simulink model "Bitchplzwork"  (Simulink 9.3)
settings: Solver=VariableStepAuto  StartTime=0.0  StopTime=1  FixedStep=0.1
values from neighbouring files (symbols this model uses):
  C = 13.5e-4    (= 0.00135)    [inverter.m]
  L = 27e-3    (= 0.027)    [inverter.m]
  R = 0.001    [inverter.m]
  Tss = 2.5e-6    (= 2.5e-06)    [inverter.m]
undefined symbols (not defined in the file or in its folder): Acid, Hydride, Lead, Metal, Nickel
libraries: powerlib x39, powerlib_extras x9, simulink x6, powerlib_meascontrol x4, electricdrivelib x2, re_lib x2, dsparch4 x1
(part 1 of 2)
settings Model: Creator=DELL  LastModifiedBy=DELL
settings Model: SuppressorTable=|
  | <?xml version="1.0" encoding="UTF-8" standalone="yes" ?>
  | <!DOCTYPE boost_serialization>
  | <boost_serialization signature="serialization::archive" version="15">
  | <DiagnosticSuppressor class_id="0" tracking_level="0" version="6">
  | 	<Table class_id="1" tracking_level="0" version="0">
  | 		<count>3</count>
  | 		<bucket_count>8</bucket_count>
  | 		<item_version>0</item_version>
  | 		<item class_id="2" tracking_level="0" version="0">
  | 			<first class_id="3" tracking_level="0" version="6">
  | 				<Source class_id="4" tracking_level="0" version="0">
  | 					<count>1</count>
  | 					<item_version>0</item_version>
  | 					<item>Bitchplzwork/PV array 1/irradiation /LimitedCounter</item>
  | 				</Source>
  | 			</first>
  | 			<second class_id="5" tracking_level="0" version="6">
  | 				<SuppressedData class_id="6" tracking_level="0" version="0">
  | 					<count>2</count>
  | 					<bucket_count>8</bucket_count>
  | 					<item_version>0</item_version>
  | 					<item class_id="7" tracking_level="0" version="0">
  | 						<first class_id="8" tracking_level="0" version="6">
  | 							<ID>Simulink:DataType:WarningOverFlowDetected</ID>
  | 							<Cause>
  | 								<Source>
  | 									<count>0</count>
  | 									<item_version>0</item_version>
  | 								</Source>
  | 							</Cause>
  | 						</first>
  | 						<second class_id="9" tracking_level="0" version="6">
  | 							<Comment></Comment>
  | 							<User></User>
  | 							<LastModified class_id="10" tracking_level="0" version="0">
  | 								<ptime_date class_id="11" tracking_level="0" version="0">
  | 									<date>20160608</date>
  | 								</ptime_date>
  | 								<ptime_time_duration class_id="12" tracking_level="0" version="0">
  | 									<is_special>0</is_special>
  | 									<time_duration_hours>15</time_duration_hours>
  | 									<time_duration_minutes>23</time_duration_minutes>
  | 									<time_duration_seconds>17</time_duration_seconds>
  | 									<time_duration_fractional_seconds>0</time_duration_fractional_seconds>
  | 								</ptime_time_duration>
  | 							</LastModified>
  | 							<SuppressionType>1</SuppressionType>
  | 						</second>
  | 					</item>
  | 					<item>
  | 						<first>
  | 							<ID>SimulinkFixedPoint:util:Overflowoccurred</ID>
  | 							<Cause>
  | 								<Source>
  | 									<count>0</count>
  | 									<item_version>0</item_version>
  | 								</Source>
  | 							</Cause>
  | 						</first>
  | 						<second>
  | 							<Comment></Comment>
  | 							<User></User>
  | 							<LastModified>
  | 								<ptime_date>
  | 									<date>20160608</date>
  | 								</ptime_date>
  | 								<ptime_time_duration>
  | 									<is_special>0</is_special>
  | 									<time_duration_hours>15</time_duration_hours>
  | 									<time_duration_minutes>23</time_duration_minutes>
  | 									<time_duration_seconds>17</time_duration_seconds>
  | 									<time_duration_fractional_seconds>0</time_duration_fractional_seconds>
  | 								</ptime_time_duration>
  | 							</LastModified>
  | 							<SuppressionType>1</SuppressionType>
  | 						</second>
  | 					</item>
  | 				</SuppressedData>
  | 			</second>
  | 		</item>
  | 		<item>
  | 			<first>
  | 				<Source>
  | 					<count>1</count>
  | 					<item_version>0</item_version>
  | 					<item>Bitchplzwork/PV array 1/Temperature/LimitedCounter</item>
  | 				</Source>
  | 			</first>
  | 			<second>
  | 				<SuppressedData>
  | 					<count>2</count>
  | 					<bucket_count>8</bucket_count>
  | 					<item_version>0</item_version>
  | 					<item>
  | 						<first>
  | 							<ID>Simulink:DataType:WarningOverFlowDetected</ID>
  | 							<Cause>
  | 								<Source>
  | 									<count>0</count>
  | 									<item_version>0</item_version>
  | 								</Source>
  | 							</Cause>
  | 						</first>
  | 						<second>
  | 							<Comment></Comment>
  | 							<User></User>
  | 							<LastModified>
  | 								<ptime_date>
  | 									<date>20160608</date>
  | 								</ptime_date>
  | 								<ptime_time_duration>
  | 									<is_special>0</is_special>
  | 									<time_duration_hours>15</time_duration_hours>
  | 									<time_duration_minutes>23</time_duration_minutes>
  | 									<time_duration_seconds>17</time_duration_seconds>
  | 									<time_duration_fractional_seconds>0</time_duration_fractional_seconds>
  | 								</ptime_time_duration>
  | 							</LastModified>
  | 							<SuppressionType>1</SuppressionType>
  | 						</second>
  | 					</item>
  | 					<item>
  | 						<first>
  | 							<ID>SimulinkFixedPoint:util:Overflowoccurred</ID>
  | 							<Cause>
  | 								<Source>
  | 									<count>0</count>
  | 									<item_version>0</item_version>
  | 								</Source>
  | 							</Cause>
  | 						</first>
  | 						<second>
  | 							<Comment></Comment>
  | 							<User></User>
  | 							<LastModified>
  | 								<ptime_date>
  | 									<date>20160608</date>
  | 								</ptime_date>
  | 								<ptime_time_duration>
  | 									<is_special>0</is_special>
  | 									<time_duration_hours>15</time_duration_hours>
  | 									<time_duration_minutes>23</time_duration_minutes>
  | 									<time_duration_seconds>17</time_duration_seconds>
  | 									<time_duration_fractional_seconds>0</time_duration_fractional_seconds>
  | 								</ptime_time_duration>
  | 							</LastModified>
  | 							<SuppressionType>1</SuppressionType>
  | 						</second>
  | 					</item>
  | 				</SuppressedData>
  | 			</second>
  | 		</item>
  | 		<item>
  | 			<first>
  | 				<Source>
  | 					<count>1</count>
  | 					<item_version>0</item_version>
  | 					<item>Bitchplzwork/Wind 3 KW, 50HZ, 440V1/Wind Speed/LimitedCounter</item>
  | 				</Source>
  | 			</first>
  | 			<second>
  | 				<SuppressedData>
  | 					<count>2</count>
  | 					<bucket_count>8</bucket_count>
  | 					<item_version>0</item_version>
  | 					<item>
  | 						<first>
  | 							<ID>Simulink:DataType:WarningOverFlowDetected</ID>
  | 							<Cause>
  | 								<Source>
  | 									<count>0</count>
  | 									<item_version>0</item_version>
  | 								</Source>
  | 							</Cause>
  | 						</first>
  | 						<second>
  | 							<Comment></Comment>
  | 							<User></User>
  | 							<LastModified>
  | 								<ptime_date>
  | 									<date>20160608</date>
  | 								</ptime_date>
  | 								<ptime_time_duration>
  | 									<is_special>0</is_special>
  | 									<time_duration_hours>15</time_duration_hours>
  | 									<time_duration_minutes>23</time_duration_minutes>
  | 									<time_duration_seconds>17</time_duration_seconds>
  | 									<time_duration_fractional_seconds>0</time_duration_fractional_seconds>
  | 								</ptime_time_duration>
  | 							</LastModified>
  | 							<SuppressionType>1</SuppressionType>
  | 						</second>
  | 					</item>
  | 					<item>
  | 						<first>
  | 							<ID>SimulinkFixedPoint:util:Overflowoccurred</ID>
  | 							<Cause>
  | 								<Source>
  | 									<count>0</count>
  | 									<item_version>0</item_version>
  | 								</Source>
  | 							</Cause>
  | 						</first>
  | 						<second>
  | 							<Comment></Comment>
  | 							<User></User>
  | 							<LastModified>
  | 								<ptime_date>
  | 									<date>20160608</date>
  | 								</ptime_date>
  | 								<ptime_time_duration>
  | 									<is_special>0</is_special>
  | 									<time_duration_hours>15</time_duration_hours>
  | 									<time_duration_minutes>23</time_duration_minutes>
  | 									<time_duration_seconds>17</time_duration_seconds>
  | 									<time_duration_fractional_seconds>0</time_duration_fractional_seconds>
  | 								</ptime_time_duration>
  | 							</LastModified>
  | 							<SuppressionType>1</SuppressionType>
  | 						</second>
  | 					</item>
  | 				</SuppressedData>
  | 			</second>
  | 		</item>
  | 	</Table>
  | </DiagnosticSuppressor>
  | </boost_serialization>
settings DataIOCC: SaveFormat=Dataset  SignalLoggingSaveFormat=Dataset  ReturnWorkspaceOutputs=on
settings OptimizationCC: LifeSpan=auto
settings DebuggingCC: UnderspecifiedInitializationDetection=Simplified  MergeDetectMultiDrivingBlocksExec=error  FcnCallInpInsideContextMsg=error  SFUnexpectedBacktrackingDiag=error  SFNoUnconditionalDefaultTransitionDiag=error  SFExecutionAtInitializationDiag=warning  ArithmeticOperatorsInVariantConditions=error
settings HardwareCC: ProdBitPerPointer=64  ProdBitPerSizeT=64  ProdBitPerPtrDiffT=64  ProdLargestAtomicFloat=Float  ProdIntDivRoundTo=Zero  ProdEndianess=LittleEndian  ProdWordSize=64  ProdHWDeviceType=Intel->x86-64 (Windows64)
settings ModelReferenceCC: PropagateSignalLabelsOutOfModel=on
settings SFSimCC: SimUseLocalCustomCode=on
settings RTWCC: RTWUseLocalCustomCode=on
settings CodeAppCC: StateflowObjectComments=off
settings GRTTargetCC: TargetLangStandard=C99 (ISO)  CombineOutputUpdateFcns=on  GRTInterface=off
settings ConfigComp: CovMetricSettings=dwe  CovHtmlReporting=off  CovSaveCumulativeToWorkspaceVar=off  CovSaveSingleToWorkspaceVar=off  CovExternalEMLEnable=on

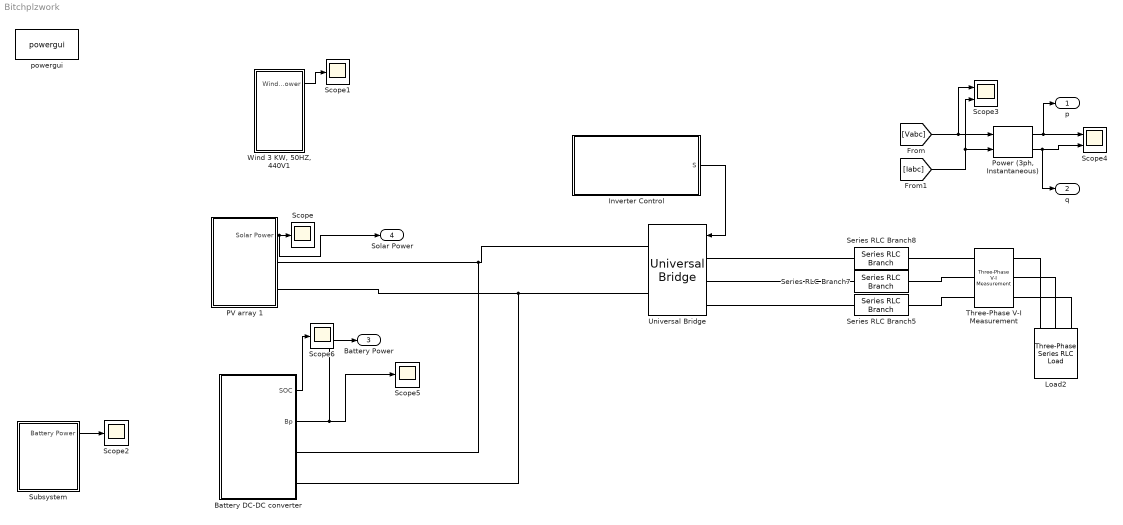
== system Bitchplzwork ==
  "Battery DC-DC converter " : Subsystem
  Inverter Control : Subsystem
  Load2 : powerlib/Elements/Three-Phase Series RLC Load  LConnTagsString=A|B|C  Configuration=Y (grounded)  NominalVoltage=400  Vabc=[1e3 1e3 1e3]  Vabcp=[1e3 1e3 1e3]  NominalFrequency=50  UnbalancedPower=off  ActivePower=400e3  InductivePower=0  CapacitivePower=0  Pabc=[10e3 9e3 11e3]  QLabc=[100 90 110]  QCabc=[100 90 110]  Pabcp=[10e3 9e3 11e3]  QLabcp=[100 90 110]  QCabcp=[100 90 110]  Measurements=None  LoadType=constant Z
      settings: SourceProductName=Simscape Electrical
  PV array 1 : Subsystem
  "Power (3ph, Instantaneous)" : powerlib_meascontrol/Measurements/Power (3ph, Instantaneous)
      settings: SourceProductName=Simscape Electrical
  Scope{,1..2,5..6} (5 alike) : Scope
  Scope3 : Scope  NumInputPorts=2
  Scope4 : Scope  NumInputPorts=2
  Series RLC Branch5 : powerlib/Elements/Series RLC Branch  LConnTagsString=__new0  RConnTagsString=__new0  BranchType=LC  Resistance=R  Inductance=L  SetiL0=off  InitialCurrent=0  Capacitance=C  Setx0=off  InitialVoltage=0  Measurements=Branch voltage
      settings: SourceProductName=Simscape Electrical
  Series RLC Branch7 : powerlib/Elements/Series RLC Branch  LConnTagsString=__new0  RConnTagsString=__new0  BranchType=LC  Resistance=R  Inductance=L  SetiL0=off  InitialCurrent=0  Capacitance=C  Setx0=off  InitialVoltage=0  Measurements=Branch voltage
      settings: SourceProductName=Simscape Electrical
  Series RLC Branch8 : powerlib/Elements/Series RLC Branch  LConnTagsString=__new0  RConnTagsString=__new0  BranchType=LC  Resistance=R  Inductance=L  SetiL0=off  InitialCurrent=0  Capacitance=C  Setx0=off  InitialVoltage=0  Measurements=Branch voltage
      settings: SourceProductName=Simscape Electrical
  Subsystem : Subsystem
  Three-Phase V-I Measurement : powerlib/Measurements/Three-Phase V-I Measurement  VoltageMeasurement=phase-to-ground  SetLabelV=on  LabelV=Vabc  Vpu=off  VpuLL=off  CurrentMeasurement=yes  SetLabelI=on  LabelI=Iabc  Ipu=off  Pbase=100e6  Vbase=500e3  OutputType=Complex  PhasorSimulation=off  PSBequivalent=0
      settings: SourceProductName=Simscape Electrical
  Universal Bridge : powerlib/Power Electronics/Universal Bridge  Arms=3  SnubberResistance=1e5  SnubberCapacitance=inf  Device=IGBT / Diodes  Ron=1e-3  Lon=0  ForwardVoltages="[  0  0  ]"  ForwardVoltage=0  GTOparameters=[ 10e-6 , 20e-6 ]  IGBTparameters=[ 1e-6 , 2e-6 ]  Measurements=None  Measurements_2=None  converterType=Rectifier
      settings: SourceProductName=Simscape Electrical
  "Wind 3 KW, 50HZ, 440V1" : Subsystem
  powergui : powerlib/powergui  Priority=1  SimulationMode=Continuous  SampleTime=Tss  frequency=60  Iterations=50  frequencyindice=0  Pbase=100e6  ErrMax=1e-4  UnitsV=kV  UnitsW=MW  buscounter=0  FunctionMessages=off  echomessages=off  EnableUseOfTLC=off  CurrentSourceSwitches=off  DisableSnubberDevices=off  DisableRonSwitches=off  DisableVfSwitches=off  DisplayEquations=off  AutomaticDiscreteSolvers=off  SolverType=Tustin/Backward Euler (TBE)  Interpol=off  ExternalGateDelay=off  methode=off  Ts=100  x0status=blocks  SPID=on  SwTol=0  HookPort=off  NonlinearTolerance=0  nMaxIteration=15  ContinueOnMaxIteration=off  RestoreLinks=warning  ResistiveCurrentMeasurement=off  Frange=[0:2:500]  Ylog=off  Xlog=on  ShowGrid=off  save=off  variable=ZData  structure=0  ZoomFFT=off  StartTime=0.0  cycles=1  DisplayStyle=1  fundamental=60  FreqAxis=off  MaxFrequency=1000  frequencyindicesteady=1  RmsSteady=1  display=off
      settings: SourceProductName=Simscape Electrical
  p : Outport
  q : Outport  Port=2
  Battery Power : Outport  Port=3
  Solar Power : Outport  Port=4
  wires:
  PV array 1/1(Solar Power) -> Solar Power/1, Scope/1
  "Wind 3 KW, 50HZ, 440V1"/1(Wind Power) -> Scope1/1
  Subsystem/1("Battery Power ") -> Scope2/1
  "Power (3ph, Instantaneous)"/2 -> q/1, Scope4/2
  "Power (3ph, Instantaneous)"/1 -> Scope4/1, p/1
  [Vabc] -> Scope3/1, "Power (3ph, Instantaneous)"/1
  [Iabc] -> Scope3/2, "Power (3ph, Instantaneous)"/2
  Inverter Control/1(S) -> Universal Bridge/1
  "Battery DC-DC converter "/2(Bp) -> Battery Power/1, Scope5/1
  "Battery DC-DC converter "/1(SOC) -> Scope6/1
  connections:
  PV array 1/RConn1 -- "Battery DC-DC converter "/RConn1 -- Universal Bridge/RConn1
  PV array 1/RConn2 -- "Battery DC-DC converter "/RConn2 -- Universal Bridge/RConn2
  Three-Phase V-I Measurement/LConn1 -- Series RLC Branch8/RConn1
  Series RLC Branch7/RConn1 -- Three-Phase V-I Measurement/LConn2
  Series RLC Branch5/RConn1 -- Three-Phase V-I Measurement/LConn3
  Three-Phase V-I Measurement/RConn1 -- Load2/LConn1
  Three-Phase V-I Measurement/RConn2 -- Load2/LConn2
  Three-Phase V-I Measurement/RConn3 -- Load2/LConn3
  Universal Bridge/LConn1 -- Series RLC Branch8/LConn1
  Universal Bridge/LConn2 -- Series RLC Branch7/LConn1
  Universal Bridge/LConn3 -- Series RLC Branch5/LConn1

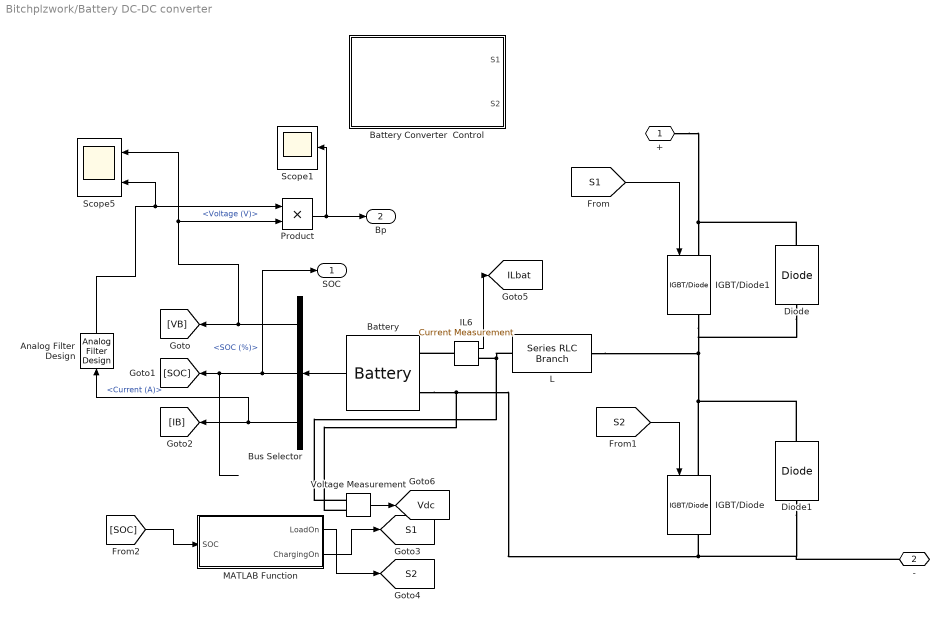
== system Bitchplzwork/Battery DC-DC converter  ==
  Analog Filter Design : dsparch4/Analog Filter Design  method=Butterworth  filttype=Lowpass  N=8  Wlo=30  Whi=80  Rp=2  Rs=40
  Battery : electricdrivelib/Extra Sources/Battery  BatType=Lead-Acid  ShowTempParam=off  ThermalPreset=no  ShowAgeParam=off  NomV=250  NomQ=500  SOC=80  Batt_Tr=30  PresetModel=on  MaxQ=520.8333  MinV=187.5  FullV=272.2039  Dis_rate=100  R=0.005  Normal_OP=155.1389  expZone="[254.523      1.666667]"  current=[6.5 13 32.5]  Units=Time  Tci=20  NomT=20  T2=-30  MaxQ2=4.8  FullV2=7.1  Normal_OP2=5.655  expZone2="[6.58           1]"  Rca=0.6  ti=2000  Dp=0  Neq0=0  Tsim=1e6  Ta1=25  Qeol=5.4*0.9  Reol=0.013333*1.2  Char_age=[2.3478, 3]  Dis_age=[2.3478, 10]  N1=1500  N2=10500  N3=1000  N4=1400  Ta2=45  N5=950
      settings: SourceProductName=Simscape Electrical
  Battery Converter  Control : Subsystem
  Bus Selector : BusSelector  OutputSignals=Voltage (V),SOC (%),Current (A)
  Diode : powerlib/Power Electronics/Diode  Ron=0.001  Lon=0  Vf=0.8  IC=0  UseSnubber=0  Rs=500  Cs=250e-9  Measurements=off
      settings: SourceProductName=Simscape Electrical
  Diode1 : powerlib/Power Electronics/Diode  Ron=0.001  Lon=0  Vf=0.8  IC=0  UseSnubber=0  Rs=500  Cs=250e-9  Measurements=off
      settings: SourceProductName=Simscape Electrical
  IGBT/Diode : powerlib/Power Electronics/IGBT//Diode  Ron=1e-3  Rs=1e5  Cs=inf  Measurements=on
      settings: SourceProductName=Simscape Electrical
  IGBT/Diode1 : powerlib/Power Electronics/IGBT//Diode  Ron=1e-3  Rs=1e5  Cs=inf  Measurements=on
      settings: SourceProductName=Simscape Electrical
  IL6 : powerlib/Measurements/Current Measurement  PhasorSimulation=off  OutputType=Complex  PSBequivalent=0
      settings: SourceProductName=Simscape Electrical
  L : powerlib/Elements/Series RLC Branch  LConnTagsString=__new0  RConnTagsString=__new0  BranchType=L  Resistance=0.1  Inductance=1e-3  SetiL0=off  InitialCurrent=0  Capacitance=1e-6  Setx0=off  InitialVoltage=0  Measurements=None
      settings: SourceProductName=Simscape Electrical
  MATLAB Function : MATLAB Function  TreatAsAtomicUnit=on
  Product : Product
  Scope1 : Scope
  Scope5 : Scope  NumInputPorts=2
  Voltage Measurement : powerlib/Measurements/Voltage Measurement  PhasorSimulation=off  OutputType=Complex  PSBequivalent=0
      settings: SourceProductName=Simscape Electrical
  + : PMIOPort  Side=Right
  - : PMIOPort  Port=2  Side=Right
  SOC : Outport
  Bp : Outport  Port=2
  tag scope: ILbat=global, S1=global, S2=global, Vdc=global
  wires:
  Bus Selector/1 -> [VB], Product/2, Scope5/1  "<Voltage (V)>"
  Product/1 -> Bp/1, Scope1/1
  Bus Selector/2 -> [SOC], SOC/1  "<SOC (%)>"
  Analog Filter Design/1 -> Scope5/2, Product/1
  Battery/1 -> Bus Selector/1
  Bus Selector/3 -> Analog Filter Design/1, [IB]  "<Current (A)>"
  [S2] -> IGBT/Diode/1
  [S1] -> IGBT/Diode1/1
  IL6/1 -> [ILbat]
  Voltage Measurement/1 -> [Vdc]
  [SOC] -> MATLAB Function/1(SOC)
  MATLAB Function/2(ChargingOn) -> [S1]
  MATLAB Function/1(LoadOn) -> [S2]
  connections:
  IL6/LConn1 -- Battery/LConn1
  Battery/LConn2 -- Voltage Measurement/LConn2 -- -/RConn1 -- Diode1/LConn1 -- IGBT/Diode/RConn1
  Diode/RConn1 -- +/RConn1 -- IGBT/Diode1/LConn1
  L/LConn1 -- Diode/LConn1 -- IGBT/Diode1/RConn1 -- Diode1/RConn1 -- IGBT/Diode/LConn1
  L/RConn1 -- Voltage Measurement/LConn1 -- IL6/RConn1

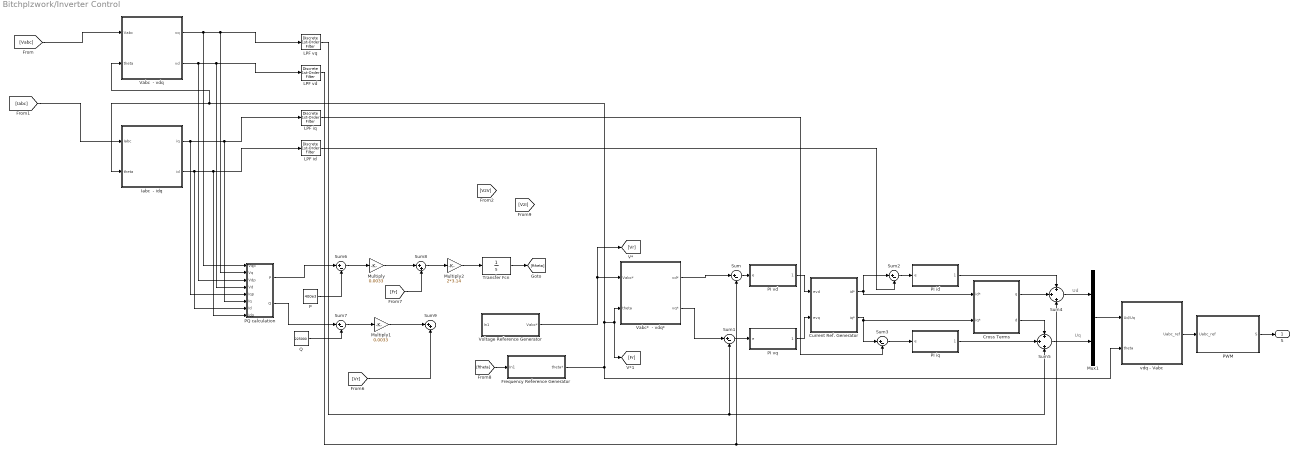
== system Bitchplzwork/Inverter Control ==
  note: Ud
  note: Uq
  " Voltage Reference Generator" : Subsystem
  Cross Terms : Subsystem
  Current Ref. Generator : Subsystem
  Frequency Reference Generator : Subsystem
  Iabc  - idq : Subsystem
  LPF id : powerlib_extras/Discrete  Control Blocks/Discrete 1st-Order Filter  FilterType=Lowpass  Tc=1e-3  Ts=5e-6  Initialize=off  Vac_Init=[0.8 -25 60]  Vdc_Init=0  PlotResponse=off  param1=[1 100 0.1]
      settings: SourceProductName=Simscape Electrical  SourceProductBaseCode=PS
  LPF iq : powerlib_extras/Discrete  Control Blocks/Discrete 1st-Order Filter  FilterType=Lowpass  Tc=1e-3  Ts=5e-6  Initialize=off  Vac_Init=[0.8 -25 60]  Vdc_Init=0  PlotResponse=off  param1=[1 100 0.1]
      settings: SourceProductName=Simscape Electrical  SourceProductBaseCode=PS
  LPF vd : powerlib_extras/Discrete  Control Blocks/Discrete 1st-Order Filter  FilterType=Lowpass  Tc=10e-3  Ts=5e-6  Initialize=off  Vac_Init=[0.8 -25 60]  Vdc_Init=-0.4  PlotResponse=off  param1=[1 100 0.1]
      settings: SourceProductName=Simscape Electrical  SourceProductBaseCode=PS
  LPF vq : powerlib_extras/Discrete  Control Blocks/Discrete 1st-Order Filter  FilterType=Lowpass  Tc=10e-3  Ts=5e-6  Initialize=off  Vac_Init=[0.8 -25 60]  Vdc_Init=0  PlotResponse=off  param1=[1 100 0.1]
      settings: SourceProductName=Simscape Electrical  SourceProductBaseCode=PS
  Multiply : Gain  Gain=0.0033
  Multiply1 : Gain  Gain=0.0033
  Multiply2 : Gain  Gain=2*3.14
  Mux1 : Mux  Inputs=2
  P : Constant  Value=400e3
  PI id : Subsystem
  PI iq : Subsystem
  PI vd : Subsystem
  PI vq : Subsystem
  PQ calculation : Subsystem
  PWM : Subsystem
  Q : Constant  Value=225000
  Sum{,1..3,6..7} (6 alike) : Sum  Inputs=|+-
  Sum4 : Sum  Inputs=+|+|+
  Sum5 : Sum  Inputs=+|+|+
  Sum8 : Sum  Inputs=|++
  Sum9 : Sum  Inputs=|++
  Transfer Fcn : TransferFcn  Denominator=[0 1 0]
  Vabc  - vdq : Subsystem
  Vabc*  - vdq* : Subsystem
  vdq - Vabc : Subsystem
  S : Outport
  wires:
  [Vabc] -> Vabc  - vdq/1(Vabc)
  [Iabc] -> Iabc  - idq/1(Iabc)
  Sum2/1 -> PI id/1(e)
  Sum3/1 -> PI iq/1(e)
  Mux1/1 -> vdq - Vabc/1(Ud/Uq)
  vdq - Vabc/1(Uabc_ref) -> PWM/1(Uabc_ref)
  PWM/1(S) -> S/1
  Vabc  - vdq/2(vd) -> PQ calculation/3(Vdp), PQ calculation/4(Vd), LPF vd/1
  Iabc  - idq/1(iq) -> PQ calculation/5(Iqp), PQ calculation/6(Iq), LPF iq/1
  Iabc  - idq/2(id) -> PQ calculation/7(Id), PQ calculation/8(Idq), LPF id/1
  LPF vd/1 -> Sum/2, Sum4/3
  LPF vq/1 -> Sum1/2, Sum5/3
  LPF iq/1 -> Sum3/2
  LPF id/1 -> Sum2/2
  Sum/1 -> PI vd/1(e)
  Sum1/1 -> PI vq/1(e)
  Vabc*  - vdq*/1(vd*) -> Sum/1
  Vabc*  - vdq*/2(vq*) -> Sum1/1
  Frequency Reference Generator/1(theta*) -> Vabc  - vdq/2(theta), Iabc  - idq/2(theta), [Fr], Vabc*  - vdq*/2(theta), vdq - Vabc/2(theta)
  PI vd/1(" ") -> Current Ref. Generator/1(evd)
  PI vq/1(" ") -> Current Ref. Generator/2(evq)
  Current Ref. Generator/2(iq*) -> Sum3/1, Cross Terms/2(iq*)
  Current Ref. Generator/1(id*) -> Cross Terms/1(id*), Sum2/1
  PI iq/1(" ") -> Sum5/2
  PI id/1(" ") -> Sum4/1
  Cross Terms/1(" q") -> Sum4/2
  Cross Terms/2(" d") -> Sum5/1
  Sum5/1 -> Mux1/2
  Sum4/1 -> Mux1/1
  Vabc  - vdq/1(vq) -> PQ calculation/1(Vqp), PQ calculation/2(Vq), LPF vq/1
  PQ calculation/1(P) -> Sum6/1
  P/1 -> Sum6/2
  Sum6/1 -> Multiply/1
  Q/1 -> Sum7/2
  PQ calculation/2(Q) -> Sum7/1
  Sum7/1 -> Multiply1/1
  Multiply/1 -> Sum8/1
  [Fr] -> Sum8/2
  Multiply1/1 -> Sum9/1
  [Vr] -> Sum9/2
  Sum8/1 -> Multiply2/1
  Multiply2/1 -> Transfer Fcn/1
  Transfer Fcn/1 -> [ftheta]
  [ftheta] -> Frequency Reference Generator/1(In1)
  " Voltage Reference Generator"/1(Vabc*) -> [Vr], Vabc*  - vdq*/1(Vabc*)

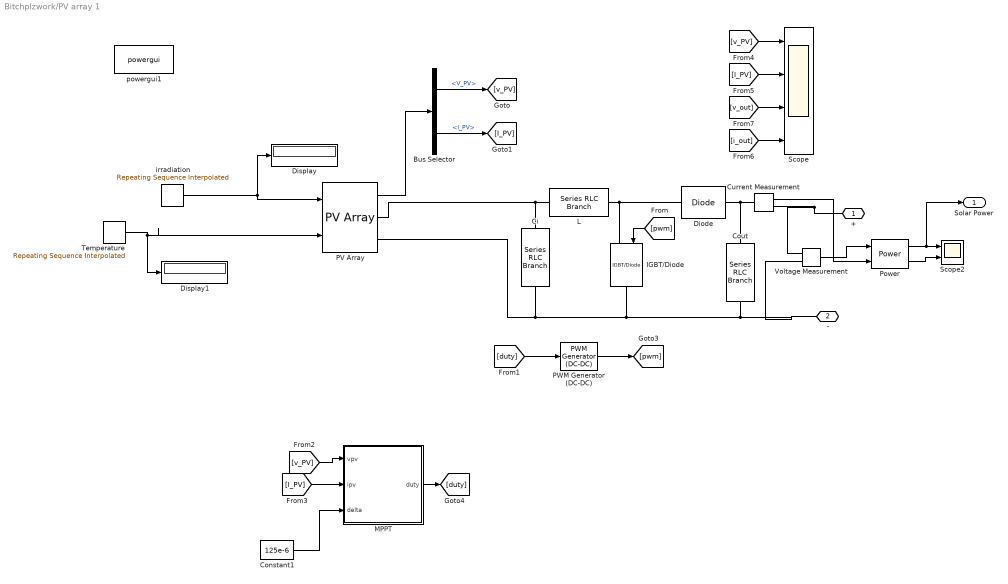
== system Bitchplzwork/PV array 1 ==
  Bus Selector : BusSelector  OutputSignals=V_PV,I_PV
  Ci : powerlib/Elements/Series RLC Branch  LConnTagsString=__new0  RConnTagsString=__new0  BranchType=RC  Resistance=1E-4  Inductance=1e-3  SetiL0=off  InitialCurrent=0  Capacitance=100E-6  Setx0=off  InitialVoltage=0  Measurements=None
      settings: SourceProductName=Simscape Electrical
  Constant1 : Constant  Value=125e-6
  Cout : powerlib/Elements/Series RLC Branch  LConnTagsString=__new0  RConnTagsString=__new0  BranchType=RC  Resistance=1E-4  Inductance=1e-3  SetiL0=off  InitialCurrent=0  Capacitance=100E-6  Setx0=off  InitialVoltage=0  Measurements=None
      settings: SourceProductName=Simscape Electrical
  Current Measurement : powerlib/Measurements/Current Measurement  PhasorSimulation=off  OutputType=Complex  PSBequivalent=0
      settings: SourceProductName=Simscape Electrical
  Diode : powerlib/Power Electronics/Diode  Ron=0.001  Lon=0  Vf=0.8  IC=0  UseSnubber=0  Rs=500  Cs=250e-9  Measurements=off
      settings: SourceProductName=Simscape Electrical
  Display : Display
  Display1 : Display
  IGBT/Diode : powerlib/Power Electronics/IGBT//Diode  Ron=1e-3  Rs=1e5  Cs=inf  Measurements=off
      settings: SourceProductName=Simscape Electrical
  L : powerlib/Elements/Series RLC Branch  LConnTagsString=__new0  RConnTagsString=__new0  BranchType=RL  Resistance=0.1  Inductance=2E-3  SetiL0=off  InitialCurrent=0  Capacitance=100E-6  Setx0=off  InitialVoltage=0  Measurements=None
      settings: SourceProductName=Simscape Electrical
  MPPT : MATLAB Function  TreatAsAtomicUnit=on
  PV Array : re_lib/Solar/PV Array  Npar=150  Nser=10  PlotType=array @ 1000 W/m2 & specified temperatures  S_vec="[ 1000  500  100 ]"  Temp_C_vec="[ 45 25  ]"  ModuleName=Shanghai JA Solar Technology JAP6-72-315-3BB  PlotWhenSelected=off  Pm=315.016  Ncell=72  Voc=46.42  Isc=8.74  Vm=37.28  Im=8.45  beta_Voc_pc=-0.3  alpha_Isc_pc=0.04  beta_Voc=-0.13926  alpha_Isc=0.003496  IL=8.9123  I0=3e-11  nI=0.95004  Rsh=1485.5559  Rs=0.45827  BAL=off  Tc=1e-6  Tfilter=5e-5
      settings: SourceProductName=Simscape Electrical
  PWM Generator (DC-DC) : powerlib_meascontrol/Pulse & Signal Generators/PWM Generator (DC-DC)  Fsw=5000  Ts=5e-6
      settings: SourceProductName=Simscape Electrical
  Power : powerlib_meascontrol/Measurements/Power  Freq=60  Vinit=[1, 0]  Iinit=[1, 0]  Ts=0
      settings: SourceProductName=Simscape Electrical
  Scope : Scope  NumInputPorts=4
  Scope2 : Scope  NumInputPorts=2
  Temperature : simulink/Sources/Repeating Sequence Interpolated  OutValues=temp  TimeValues=timeStamp  LookUpMeth=Interpolation-Use End Values  tsamp=0.1  OutMin=[]  OutMax=[]  OutDataTypeStr=double  OutputDataTypeScalingMode=double  OutDataType=fixdt(0,8)  OutScaling=2^-10
  Voltage Measurement : powerlib/Measurements/Voltage Measurement  PhasorSimulation=off  OutputType=Complex  PSBequivalent=0
      settings: SourceProductName=Simscape Electrical
  "irradiation " : simulink/Sources/Repeating Sequence Interpolated  OutValues=irrad  TimeValues=timeStamp  LookUpMeth=Interpolation-Use End Values  tsamp=0.1  OutMin=[]  OutMax=[]  OutDataTypeStr=double  OutputDataTypeScalingMode=double  OutDataType=fixdt(0,8)  OutScaling=2^-10
  powergui1 : powerlib/powergui  Priority=1  SimulationMode=Discrete  SampleTime=Tss  frequency=60  Iterations=50  frequencyindice=0  Pbase=100e6  ErrMax=1e-4  UnitsV=kV  UnitsW=MW  buscounter=0  FunctionMessages=off  echomessages=off  EnableUseOfTLC=off  CurrentSourceSwitches=off  DisableSnubberDevices=off  DisableRonSwitches=off  DisableVfSwitches=off  DisplayEquations=off  AutomaticDiscreteSolvers=off  SolverType=Tustin/Backward Euler (TBE)  Interpol=off  ExternalGateDelay=off  methode=off  Ts=100  x0status=blocks  SPID=on  SwTol=0  HookPort=off  NonlinearTolerance=0  nMaxIteration=15  ContinueOnMaxIteration=off  RestoreLinks=warning  ResistiveCurrentMeasurement=off  Frange=[0:2:500]  Ylog=off  Xlog=on  ShowGrid=off  save=off  variable=ZData  structure=0  ZoomFFT=off  StartTime=0.0  cycles=1  DisplayStyle=1  fundamental=60  FreqAxis=off  MaxFrequency=1000  frequencyindicesteady=1  RmsSteady=1  display=off
      settings: SourceProductName=Simscape Electrical
  + : PMIOPort  Side=Right
  - : PMIOPort  Port=2  Side=Right
  Solar Power : Outport
  wires:
  Bus Selector/1 -> [v_PV]  "<V_PV>"
  Bus Selector/2 -> [I_PV]  "<I_PV>"
  MPPT/1(duty) -> [duty]
  Constant1/1 -> MPPT/3(delta)
  [i_out] -> Scope/4
  "irradiation "/1 -> PV Array/1, Display/1
  [duty] -> PWM Generator (DC-DC)/1
  PWM Generator (DC-DC)/1 -> [pwm]
  PV Array/1 -> Bus Selector/1
  [v_out] -> Scope/3
  [I_PV] -> Scope/2
  [v_PV] -> Scope/1
  Temperature/1 -> PV Array/2, Display1/1
  Power/2 -> Scope2/2
  Power/1 -> Solar Power/1, Scope2/1
  [pwm] -> IGBT/Diode/1
  Voltage Measurement/1 -> Power/1
  Current Measurement/1 -> Power/2
  [v_PV] -> MPPT/1(vpv)
  [I_PV] -> MPPT/2(ipv)
  connections:
  Diode/RConn1 -- Cout/LConn1 -- Current Measurement/LConn1
  PV Array/RConn1 -- L/LConn1 -- Ci/LConn1
  Cout/RConn1 -- PV Array/RConn2 -- Ci/RConn1 -- IGBT/Diode/RConn1 -- Voltage Measurement/LConn2 -- -/RConn1
  Diode/LConn1 -- IGBT/Diode/LConn1 -- L/RConn1
  Current Measurement/RConn1 -- +/RConn1 -- Voltage Measurement/LConn1

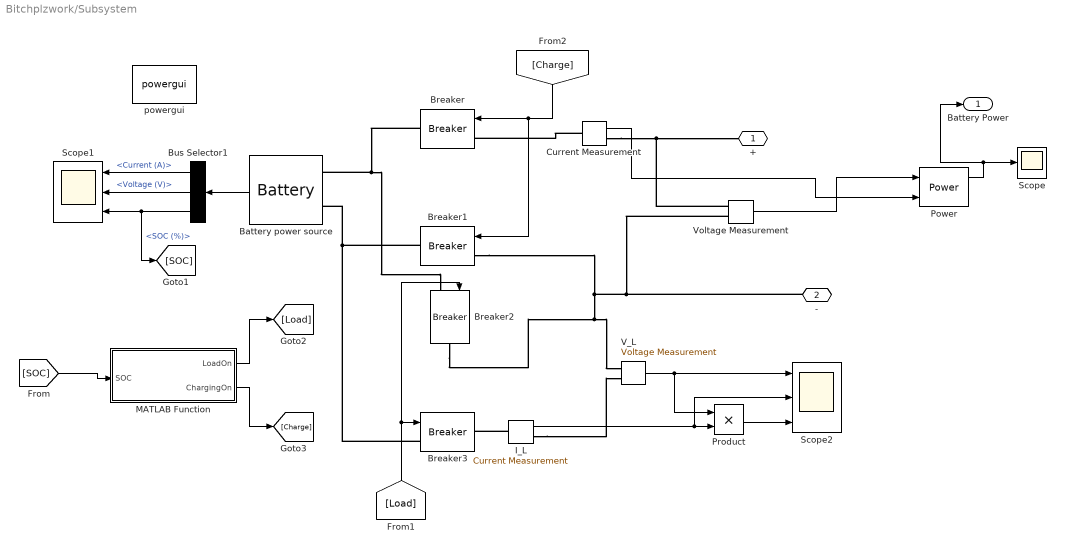
== system Bitchplzwork/Subsystem ==
  Battery power source : electricdrivelib/Extra Sources/Battery  BatType=Nickel-Metal-Hydride  ShowTempParam=off  ThermalPreset=no  ShowAgeParam=off  NomV=100  NomQ=1.5  SOC=80  Batt_Tr=30  PresetModel=on  MaxQ=1.6154  MinV=75  FullV=117.7966  Dis_rate=0.3  R=0.66667  Normal_OP=1.4423  expZone="[108.4746           0.3]"  current=[1.5 3]  Units=Ampere-hour  Tci=20  NomT=25  T2=0  MaxQ2=2.208  FullV2=3.45  Normal_OP2=2.8  expZone2="[3.22        0.23]"  Rca=0.6  ti=1000  Dp=0  Neq0=0  Tsim=1e6  Ta1=25  Qeol=5.4*0.9  Reol=0.013333*1.2  Char_age=[2.3478, 3]  Dis_age=[2.3478, 10]  N1=1500  N2=10500  N3=1000  N4=1400  Ta2=45  N5=950
      settings: SourceProductName=Simscape Electrical
  Breaker{,1..3} (4 alike) : powerlib/Elements/Breaker  InitialState=0  SwitchingTimes="[ 1/60  5/60 ]"  External=on  BreakerResistance=0.01  SnubberResistance=1e6  SnubberCapacitance=inf  Measurements=None  MoreParameters=off  NoBreakLoop=off
      settings: SourceProductName=Simscape Electrical
  Bus Selector1 : BusSelector  OutputSignals=Current (A),Voltage (V),SOC (%)
  Current Measurement : powerlib/Measurements/Current Measurement  PhasorSimulation=off  OutputType=Complex  PSBequivalent=0
      settings: SourceProductName=Simscape Electrical
  I_L : powerlib/Measurements/Current Measurement  PhasorSimulation=off  OutputType=Complex  PSBequivalent=0
      settings: SourceProductName=Simscape Electrical
  MATLAB Function : MATLAB Function  TreatAsAtomicUnit=on
  Power : powerlib_meascontrol/Measurements/Power  Freq=60  Vinit=[1, 0]  Iinit=[1, 0]  Ts=0
      settings: SourceProductName=Simscape Electrical
  Product : Product  RndMeth=Zero
  Scope : Scope
  Scope1 : Scope  NumInputPorts=3
  Scope2 : Scope  NumInputPorts=3
  V_L : powerlib/Measurements/Voltage Measurement  PhasorSimulation=off  OutputType=Complex  PSBequivalent=0
      settings: SourceProductName=Simscape Electrical
  Voltage Measurement : powerlib/Measurements/Voltage Measurement  PhasorSimulation=off  OutputType=Complex  PSBequivalent=0
      settings: SourceProductName=Simscape Electrical
  powergui : powerlib/powergui  Priority=1  SimulationMode=Continuous  SampleTime=50e-6  frequency=60  Iterations=50  frequencyindice=0  Pbase=100e6  ErrMax=1e-4  UnitsV=kV  UnitsW=MW  buscounter=0  FunctionMessages=off  echomessages=off  EnableUseOfTLC=off  CurrentSourceSwitches=on  DisableSnubberDevices=off  DisableRonSwitches=off  DisableVfSwitches=off  DisplayEquations=off  AutomaticDiscreteSolvers=off  SolverType=Tustin  Interpol=off  ExternalGateDelay=off  methode=off  Ts=10  x0status=blocks  SPID=off  SwTol=0  HookPort=off  NonlinearTolerance=0  nMaxIteration=15  ContinueOnMaxIteration=off  RestoreLinks=warning  ResistiveCurrentMeasurement=off  Frange=[0:2:500]  Ylog=off  Xlog=on  ShowGrid=off  save=off  variable=ZData  structure=0  ZoomFFT=off  StartTime=0.0  cycles=1  DisplayStyle=1  fundamental=60  FreqAxis=off  MaxFrequency=1000  frequencyindicesteady=1  RmsSteady=1  display=off
      settings: SourceProductName=Simscape Electrical
  + : PMIOPort  Side=Right
  - : PMIOPort  Port=2  Side=Right
  "Battery Power " : Outport
  wires:
  Bus Selector1/1 -> Scope1/1  "<Current (A)>"
  [Load] -> Breaker3/1, Breaker2/1
  [Charge] -> Breaker/1, Breaker1/1
  MATLAB Function/2(ChargingOn) -> [Charge]
  MATLAB Function/1(LoadOn) -> [Load]
  Bus Selector1/3 -> Scope1/3, [SOC]  "<SOC (%)>"
  [SOC] -> MATLAB Function/1(SOC)
  Product/1 -> Scope2/3
  V_L/1 -> Scope2/1, Product/1
  I_L/1 -> Scope2/2, Product/2
  Battery power source/1 -> Bus Selector1/1
  Bus Selector1/2 -> Scope1/2  "<Voltage (V)>"
  Voltage Measurement/1 -> Power/1
  Current Measurement/1 -> Power/2
  Power/1 -> Scope/1, "Battery Power "/1
  connections:
  Breaker2/LConn1 -- Breaker/RConn1 -- Battery power source/LConn1
  Voltage Measurement/LConn1 -- Current Measurement/RConn1 -- +/RConn1
  Breaker1/RConn1 -- Breaker3/LConn1 -- Battery power source/LConn2
  I_L/RConn1 -- V_L/LConn2
  V_L/LConn1 -- Voltage Measurement/LConn2 -- -/RConn1 -- Breaker1/LConn1 -- Breaker2/RConn1
  I_L/LConn1 -- Breaker3/RConn1
  Current Measurement/LConn1 -- Breaker/LConn1

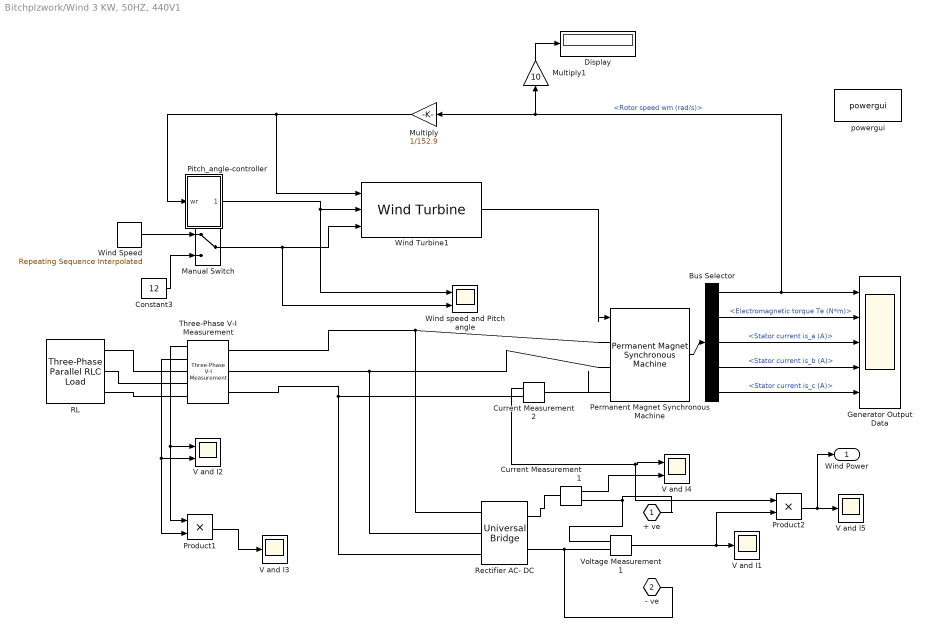
== system Bitchplzwork/Wind 3 KW, 50HZ, 440V1 ==
  Bus Selector : BusSelector  OutputSignals=Rotor speed wm (rad/s),Electromagnetic torque Te (N*m),Stator current is_a (A),Stator current is_b (A),Stator current is_c (A)
  Constant3 : Constant  Value=12
  Current Measurement1 : powerlib/Measurements/Current Measurement  PhasorSimulation=off  OutputType=Complex  PSBequivalent=0
      settings: SourceProductName=Simscape Electrical
  Current Measurement2 : powerlib/Measurements/Current Measurement  PhasorSimulation=off  OutputType=Complex  PSBequivalent=0
      settings: SourceProductName=Simscape Electrical
  Display : Display
  Generator Output Data : Scope  NumInputPorts=5
  Manual Switch : ManualSwitch
  Multiply : Gain  Gain=1/152.9
  Multiply1 : Gain  Gain=10
  Permanent Magnet Synchronous Machine : powerlib/Machines/Permanent Magnet Synchronous Machine  NbPhases=3  FluxDistribution=Sinusoidal  RotorType=Round  MechanicalLoad=Torque Tm  PresetModel="05:  8 Nm 300 Vdc 2000 RPM - 10 Nm"  ShowDetailedParameters=on  MeasurementBus=off  Resistance=0.9585  Inductance=8.5e-3  dqInductances=[8.5e-3,8.5e-3]  La=0.00525  MachineConstant=Flux linkage established by magnets (V.s)  Flux=0.1827  VoltageCst=132.5525  TorqueCst=1.0962  Flat=120  Mechanical=[0.0006329 0.0003035 4 0]  PolePairs=4  InitialConditions=[0,0, 0,0]  InitialConditions5ph=[0 0 0 0 0 0]  TsPowergui=0  TsBlock=-1  RefAngle=90 degrees behind phase A axis (modified Park)
  Pitch_angle-controller : Subsystem
  Product1 : Product
  Product2 : Product
  "RL " : powerlib/Elements/Three-Phase Parallel RLC Load  LConnTagsString=A|B|C  Configuration=Y (grounded)  NominalVoltage=400  Vabc=[1e3 1e3 1e3]  Vabcp=[1e3 1e3 1e3]  NominalFrequency=50  UnbalancedPower=off  ActivePower=0  InductivePower=0  CapacitivePower=400e3  Pabc=[10e3 9e3 11e3]  QLabc=[100 90 110]  QCabc=[100 90 110]  Pabcp=[10e3 9e3 11e3]  QLabcp=[100 90 110]  QCabcp=[100 90 110]  Measurements=None  LoadType=constant Z
      settings: SourceProductName=Simscape Electrical
  Rectifier AC- DC : powerlib/Power Electronics/Universal Bridge  Arms=3  SnubberResistance=1e5  SnubberCapacitance=inf  Device=Diodes  Ron=1e-3  Lon=0  ForwardVoltages="[  0  0  ]"  ForwardVoltage=0.1  GTOparameters=[ 10e-6 , 20e-6 ]  IGBTparameters=[ 1e-6 , 2e-6 ]  Measurements=None  Measurements_2=None  converterType=Rectifier
      settings: SourceProductName=Simscape Electrical
  Three-Phase V-I Measurement : powerlib/Measurements/Three-Phase V-I Measurement  VoltageMeasurement=phase-to-ground  SetLabelV=off  LabelV=Vabc  Vpu=off  VpuLL=off  CurrentMeasurement=yes  SetLabelI=off  LabelI=Iabc  Ipu=off  Pbase=100e6  Vbase=500e3  OutputType=Complex  PhasorSimulation=off  PSBequivalent=0
      settings: SourceProductName=Simscape Electrical
  V and I1 : Scope
  V and I2 : Scope  NumInputPorts=2
  V and I3 : Scope
  V and I4 : Scope  NumInputPorts=2
  V and I5 : Scope
  Voltage Measurement1 : powerlib/Measurements/Voltage Measurement  PhasorSimulation=off  OutputType=Complex  PSBequivalent=0
      settings: SourceProductName=Simscape Electrical
  Wind Speed : simulink/Sources/Repeating Sequence Interpolated  OutValues=temp  TimeValues=timeStamp  LookUpMeth=Interpolation-Use End Values  tsamp=0.1  OutMin=[]  OutMax=[]  OutDataTypeStr=double  OutputDataTypeScalingMode=double  OutDataType=fixdt(0,8)  OutScaling=2^-10
  Wind Turbine1 : re_lib/Wind Generation/Wind Turbine  Pnom=1.5e6  Pelec_base=1.5e6/.9  wind_base=12  P_wind_base=0.8  speed_nom=1.2  pitch_angle=0  c1_c6="[0.51763          116          0.4            5           21     0.006795]"  cp_nom=0.48  lambda_nom=8.1
      settings: SourceProductName=Simscape Electrical  SourceProductBaseCode=PS
  Wind speed and Pitch angle : Scope  NumInputPorts=2
  powergui : powerlib/powergui  Priority=1  SimulationMode=Continuous  SampleTime=50e-6  frequency=60  Iterations=50  frequencyindice=60  Pbase=100e6  ErrMax=1e-4  UnitsV=kV  UnitsW=MW  buscounter=0  FunctionMessages=off  echomessages=off  EnableUseOfTLC=off  CurrentSourceSwitches=off  DisableSnubberDevices=off  DisableRonSwitches=off  DisableVfSwitches=off  DisplayEquations=off  AutomaticDiscreteSolvers=off  SolverType=Tustin/Backward Euler (TBE)  Interpol=off  ExternalGateDelay=off  methode=off  Ts=100  x0status=blocks  SPID=on  SwTol=0  HookPort=off  NonlinearTolerance=0  nMaxIteration=15  ContinueOnMaxIteration=off  RestoreLinks=warning  ResistiveCurrentMeasurement=off  Frange=[0:2:500]  Ylog=off  Xlog=on  ShowGrid=off  save=off  variable=ZData  structure=0  ZoomFFT=off  StartTime=0.0  cycles=1  DisplayStyle=1  fundamental=60  FreqAxis=off  MaxFrequency=1000  frequencyindicesteady=1  RmsSteady=1  display=off
      settings: SourceProductName=Simscape Electrical
  + ve : PMIOPort  Side=Right
  - ve : PMIOPort  Port=2  Side=Right
  Wind Power : Outport
  wires:
  Product2/1 -> V and I5/1, Wind Power/1
  Current Measurement2/1 -> V and I4/1, Product2/1
  Voltage Measurement1/1 -> V and I1/1, Product2/2
  Product1/1 -> V and I3/1
  Three-Phase V-I Measurement/2 -> V and I2/2, Product1/2
  Three-Phase V-I Measurement/1 -> V and I2/1, Product1/1
  Manual Switch/1 -> Wind speed and Pitch angle/2, Wind Turbine1/3
  Constant3/1 -> Manual Switch/2
  Wind Speed/1 -> Manual Switch/1
  Bus Selector/5 -> Generator Output Data/5  "<Stator current is_c (A)>"
  Bus Selector/4 -> Generator Output Data/4  "<Stator current is_b (A)>"
  Bus Selector/3 -> Generator Output Data/3  "<Stator current is_a (A)>"
  Bus Selector/2 -> Generator Output Data/2  "<Electromagnetic torque Te (N*m)>"
  Bus Selector/1 -> Multiply1/1, Multiply/1, Generator Output Data/1  "<Rotor speed wm (rad/s)>"
  Permanent Magnet Synchronous Machine/1 -> Bus Selector/1
  Multiply/1 -> Wind Turbine1/1, Pitch_angle-controller/1(wr)
  Pitch_angle-controller/1(Pitch_angle) -> Wind speed and Pitch angle/1, Wind Turbine1/2
  Wind Turbine1/1 -> Permanent Magnet Synchronous Machine/1
  Current Measurement1/1 -> V and I4/2
  Multiply1/1 -> Display/1
  connections:
  "RL "/LConn3 -- Three-Phase V-I Measurement/RConn3
  Three-Phase V-I Measurement/RConn2 -- "RL "/LConn2
  "RL "/LConn1 -- Three-Phase V-I Measurement/RConn1
  Current Measurement2/LConn1 -- Permanent Magnet Synchronous Machine/LConn3
  Current Measurement1/LConn1 -- Rectifier AC- DC/RConn1
  + ve/RConn1 -- Voltage Measurement1/LConn1 -- Current Measurement1/RConn1
  Rectifier AC- DC/RConn2 -- - ve/RConn1 -- Voltage Measurement1/LConn2
  Permanent Magnet Synchronous Machine/LConn1 -- Rectifier AC- DC/LConn1 -- Three-Phase V-I Measurement/LConn1
  Current Measurement2/RConn1 -- Three-Phase V-I Measurement/LConn3 -- Rectifier AC- DC/LConn3
  Permanent Magnet Synchronous Machine/LConn2 -- Rectifier AC- DC/LConn2 -- Three-Phase V-I Measurement/LConn2

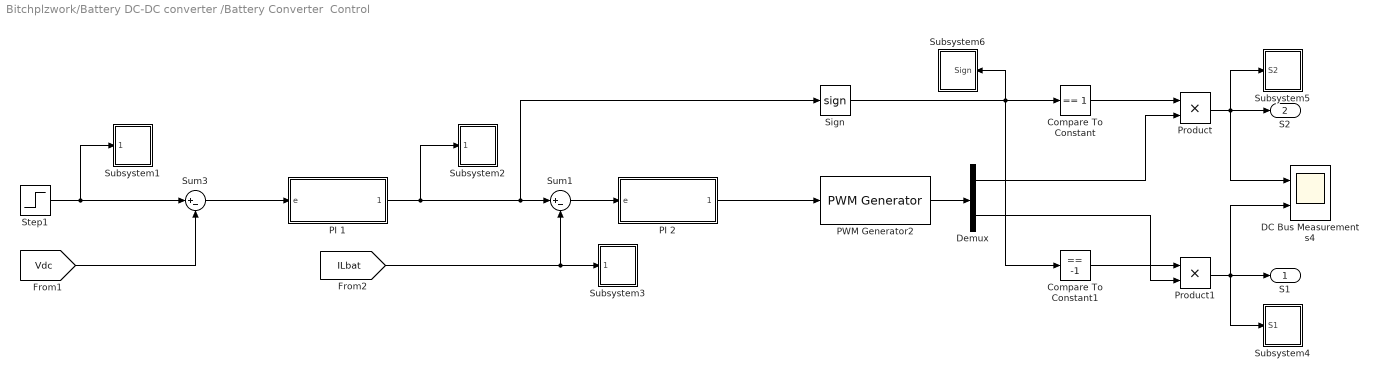
== system Bitchplzwork/Battery DC-DC converter /Battery Converter  Control ==
  Compare To Constant : simulink/Logic and Bit Operations/Compare To Constant  relop===  const=1  OutDataTypeStr=uint8
  Compare To Constant1 : simulink/Logic and Bit Operations/Compare To Constant  relop===  const=-1  OutDataTypeStr=uint8
  DC Bus Measurements4 : Scope  NumInputPorts=2
  Demux : Demux  Outputs=2
  PI 1 : Subsystem
  PI 2 : Subsystem
  PWM Generator2 : powerlib_extras/Control  Blocks/PWM Generator  GeneratorMode="1-arm  bridge (2 pulses)"  Fc=10000  Internal=off  mIndex=0.2  Freq=0  Phase=0
      link override Triangle: rep_seq_y=[0 1 0]  rep_seq_t=[0 1/Fc/2 1/Fc]
      settings: SourceProductName=Simscape Electrical  SourceProductBaseCode=PS
  Product : Product  RndMeth=Zero
  Product1 : Product  RndMeth=Zero
  Sign : Signum  SampleTime=5e-6
  Step1 : Step  Time=0  After=1000  SampleTime=0
  Subsystem1 : Subsystem
  Subsystem2 : Subsystem
  Subsystem3 : Subsystem
  Subsystem4 : Subsystem
  Subsystem5 : Subsystem
  Subsystem6 : Subsystem
  Sum1 : Sum  Inputs=|+-
  Sum3 : Sum  Inputs=|+-
  S1 : Outport
  S2 : Outport  Port=2
  wires:
  Step1/1 -> Sum3/1, Subsystem1/1(Vdc_ref)
  Sum3/1 -> PI 1/1(e)
  Sum1/1 -> PI 2/1(e)
  [ILbat] -> Sum1/2, Subsystem3/1(ILbat)
  PI 1/1(" ") -> Sum1/1, Sign/1, Subsystem2/1(Ibat_ref)
  PI 2/1(" ") -> PWM Generator2/1
  PWM Generator2/1 -> Demux/1
  Sign/1 -> Compare To Constant/1, Compare To Constant1/1, Subsystem6/1(Sign)
  Compare To Constant/1 -> Product/1
  Demux/1 -> Product/2
  Compare To Constant1/1 -> Product1/1
  Product/1 -> DC Bus Measurements4/1, S2/1, Subsystem5/1(S2)
  Product1/1 -> S1/1, Subsystem4/1(S1), DC Bus Measurements4/2
  Demux/2 -> Product1/2
  [Vdc] -> Sum3/2

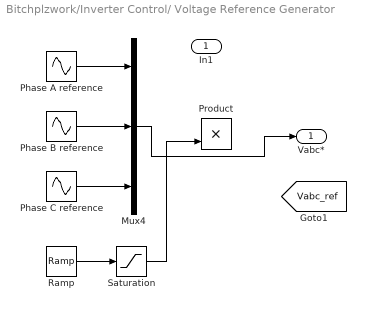
== system Bitchplzwork/Inverter Control/ Voltage Reference Generator ==
  In1 : Inport
  Mux4 : Mux  Inputs=3
  Phase A reference : Sin  Amplitude=400*sqrt(2)/sqrt(3)  Frequency=2*pi*50  SampleTime=0
  Phase B reference : Sin  Amplitude=400*sqrt(2)/sqrt(3)  Frequency=2*pi*50  Phase=-2*pi/3  SampleTime=0
  Phase C reference : Sin  Amplitude=400*sqrt(2)/sqrt(3)  Frequency=2*pi*50  Phase=2*pi/3  SampleTime=0
  Product : Product  RndMeth=Zero
  Ramp : simulink/Sources/Ramp  slope=1/0.3  start=0  InitialOutput=0
  Saturation : Saturate  UpperLimit=1  LowerLimit=0
  Vabc* : Outport
  tag scope: Vabc_ref=global
  wires:
  Phase B reference/1 -> Mux4/2
  Phase A reference/1 -> Mux4/1
  Phase C reference/1 -> Mux4/3
  Ramp/1 -> Saturation/1
  Saturation/1 -> Product/2
  Mux4/1 -> Vabc*/1

== system Bitchplzwork/Inverter Control/Cross Terms ==
  id* : Inport
  iq* : Inport  Port=2
  Gain1 : Gain  Gain=-2*pi*50*3e-3
  Gain2 : Gain  Gain=2*pi*50*3e-3
  " q" : Outport
  " d" : Outport  Port=2
  wires:
  id*/1 -> Gain1/1
  iq*/1 -> Gain2/1
  Gain1/1 -> " d"/1
  Gain2/1 -> " q"/1

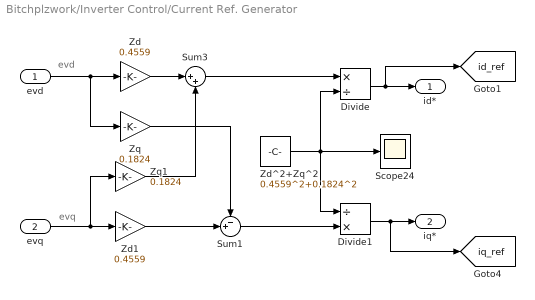
== system Bitchplzwork/Inverter Control/Current Ref. Generator ==
  note: evd
  note: evq
  evd : Inport
  evq : Inport  Port=2
  Divide : Product  Inputs=*/
  Divide1 : Product  Inputs=/*
  Scope24 : Scope
  Sum1 : Sum  Inputs=-+|
  Sum3 : Sum  Inputs=|++
  Zd : Gain  Gain=0.4559
  Zd1 : Gain  Gain=0.4559
  Zd^2+Zq^2 : Constant  Value=0.4559^2+0.1824^2
  Zq : Gain  Gain=0.1824
  Zq1 : Gain  Gain=0.1824
  id* : Outport
  iq* : Outport  Port=2
  tag scope: id_ref=global, iq_ref=global
  wires:
  Zd/1 -> Sum3/1
  Zq1/1 -> Sum3/2
  Zd1/1 -> Sum1/2
  Zq/1 -> Sum1/1
  Sum3/1 -> Divide/1
  Zd^2+Zq^2/1 -> Divide/2, Divide1/1, Scope24/1
  Sum1/1 -> Divide1/2
  evd/1 -> Zd/1, Zq/1
  evq/1 -> Zd1/1, Zq1/1
  Divide1/1 -> iq*/1, [iq_ref]
  Divide/1 -> id*/1, [id_ref]

== system Bitchplzwork/Inverter Control/Frequency Reference Generator ==
  note: theta
  In1 : Inport
  Constant : Constant  Value=2*pi
  Integrator : Integrator  ExternalReset=rising
  Relational Operator : RelationalOperator  OutDataTypeStr=boolean  RndMeth=Nearest
  w* : Gain  Gain=2*pi
  theta* : Outport
  tag scope: f_ref=global, theta=global
  wires:
  w*/1 -> Integrator/1
  Relational Operator/1 -> Integrator/2
  Constant/1 -> Relational Operator/2
  Integrator/1 -> Relational Operator/1, theta*/1, [theta]
  In1/1 -> [f_ref], w*/1

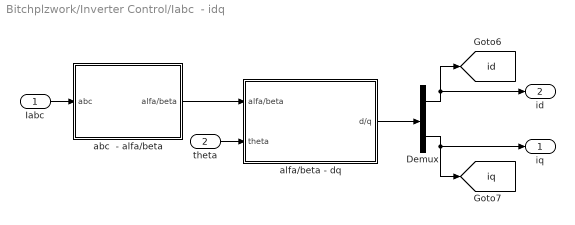
== system Bitchplzwork/Inverter Control/Iabc  - idq ==
  Iabc : Inport
  theta : Inport  Port=2
  Demux : Demux  Outputs=2
  abc  - alfa/beta : Subsystem
  alfa/beta - dq : Subsystem
  iq : Outport
  id : Outport  Port=2
  tag scope: id=global, iq=global
  wires:
  theta/1 -> alfa/beta - dq/2(theta)
  Iabc/1 -> abc  - alfa/beta/1(abc)
  abc  - alfa/beta/1(alfa/beta) -> alfa/beta - dq/1(alfa/beta)
  alfa/beta - dq/1(d/q) -> Demux/1
  Demux/1 -> id/1, [id]
  Demux/2 -> iq/1, [iq]

== system Bitchplzwork/Inverter Control/PI id ==
  e : Inport
  Gain1 : Gain  Gain=50
  Gain2 : Gain  Gain=500
  Integrator : Integrator
  Saturation : Saturate  UpperLimit=inf  LowerLimit=-inf
  Sum1 : Sum  Inputs=|++
  " " : Outport
  wires:
  Sum1/1 -> Saturation/1
  Integrator/1 -> Sum1/2
  Gain1/1 -> Sum1/1
  e/1 -> Gain2/1, Gain1/1
  Gain2/1 -> Integrator/1
  Saturation/1 -> " "/1

== system Bitchplzwork/Inverter Control/PI iq ==
  e : Inport
  Gain1 : Gain  Gain=50
  Gain2 : Gain  Gain=500
  Integrator : Integrator
  Saturation : Saturate  UpperLimit=inf  LowerLimit=-inf
  Sum1 : Sum  Inputs=|++
  " " : Outport
  wires:
  Saturation/1 -> " "/1
  Gain2/1 -> Integrator/1
  e/1 -> Gain1/1, Gain2/1
  Gain1/1 -> Sum1/1
  Integrator/1 -> Sum1/2
  Sum1/1 -> Saturation/1

== system Bitchplzwork/Inverter Control/PI vd ==
  e : Inport
  Gain1 : Gain  Gain=2
  Gain2 : Gain  Gain=20
  Integrator : Integrator
  Saturation : Saturate  UpperLimit=inf  LowerLimit=-inf
  Sum1 : Sum  Inputs=|++
  " " : Outport
  wires:
  Saturation/1 -> " "/1
  Gain2/1 -> Integrator/1
  e/1 -> Gain1/1, Gain2/1
  Gain1/1 -> Sum1/1
  Integrator/1 -> Sum1/2
  Sum1/1 -> Saturation/1

== system Bitchplzwork/Inverter Control/PI vq ==
  e : Inport
  Gain1 : Gain  Gain=2
  Gain2 : Gain  Gain=2
  Integrator : Integrator
  Saturation : Saturate  UpperLimit=inf  LowerLimit=-inf
  Sum1 : Sum  Inputs=|++
  " " : Outport
  wires:
  Sum1/1 -> Saturation/1
  Integrator/1 -> Sum1/2
  Gain1/1 -> Sum1/1
  e/1 -> Gain2/1, Gain1/1
  Gain2/1 -> Integrator/1
  Saturation/1 -> " "/1

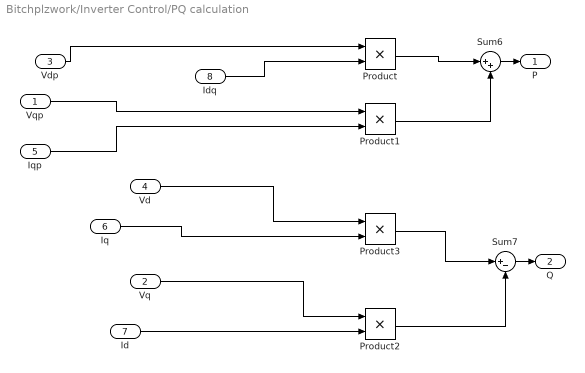
== system Bitchplzwork/Inverter Control/PQ calculation ==
  Vqp : Inport
  Vq : Inport  Port=2
  Vdp : Inport  Port=3
  Vd : Inport  Port=4
  Iqp : Inport  Port=5
  Iq : Inport  Port=6
  Id : Inport  Port=7
  Idq : Inport  Port=8
  Product{,1..3} (4 alike) : Product
  Sum6 : Sum  Inputs=|++
  Sum7 : Sum  Inputs=|+-
  P : Outport
  Q : Outport  Port=2
  wires:
  Sum6/1 -> P/1
  Product3/1 -> Sum7/1
  Product1/1 -> Sum6/2
  Product/1 -> Sum6/1
  Vq/1 -> Product2/1
  Sum7/1 -> Q/1
  Product2/1 -> Sum7/2
  Iqp/1 -> Product1/2
  Vd/1 -> Product3/1
  Id/1 -> Product2/2
  Vdp/1 -> Product/1
  Idq/1 -> Product/2
  Vqp/1 -> Product1/1
  Iq/1 -> Product3/2

== system Bitchplzwork/Inverter Control/PWM ==
  Uabc_ref : Inport
  Gain2 : Gain  Gain=2/1000
  PWM Generator : powerlib_extras/Control  Blocks/PWM Generator  GeneratorMode="3-arm  bridge (6 pulses)"  Fc=10000  Internal=off  mIndex=0.4  Freq=60  Phase=0
      settings: SourceProductName=Simscape Electrical  SourceProductBaseCode=PS
  S : Outport
  tag scope: m_index=global, pulses=global
  wires:
  PWM Generator/1 -> S/1, [pulses]
  Uabc_ref/1 -> Gain2/1
  Gain2/1 -> PWM Generator/1, [m_index]

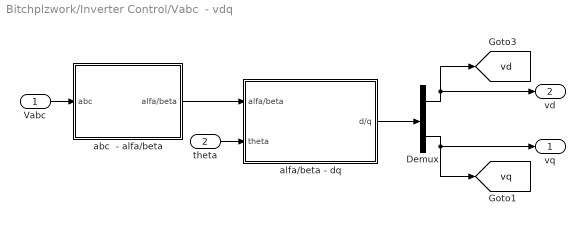
== system Bitchplzwork/Inverter Control/Vabc  - vdq ==
  Vabc : Inport
  theta : Inport  Port=2
  Demux : Demux  Outputs=2
  abc  - alfa/beta : Subsystem
  alfa/beta - dq : Subsystem
  vq : Outport
  vd : Outport  Port=2
  tag scope: vd=global, vq=global
  wires:
  Demux/2 -> vq/1, [vq]
  Demux/1 -> vd/1, [vd]
  alfa/beta - dq/1(d/q) -> Demux/1
  abc  - alfa/beta/1(alfa/beta) -> alfa/beta - dq/1(alfa/beta)
  Vabc/1 -> abc  - alfa/beta/1(abc)
  theta/1 -> alfa/beta - dq/2(theta)

== system Bitchplzwork/Inverter Control/Vabc*  - vdq* ==
  Vabc* : Inport
  theta : Inport  Port=2
  Demux : Demux  Outputs=2
  abc  - alfa/beta : Subsystem
  alfa/beta - dq : Subsystem
  vd* : Outport
  vq* : Outport  Port=2
  tag scope: vd_ref=global, vq_ref=global
  wires:
  theta/1 -> alfa/beta - dq/2(theta)
  Vabc*/1 -> abc  - alfa/beta/1(abc)
  abc  - alfa/beta/1(alfa/beta) -> alfa/beta - dq/1(alfa/beta)
  alfa/beta - dq/1(d/q) -> Demux/1
  Demux/1 -> vd*/1, [vd_ref]
  Demux/2 -> vq*/1, [vq_ref]

== system Bitchplzwork/Inverter Control/vdq - Vabc ==
  Ud/Uq : Inport
  theta : Inport  Port=2
  alfa/beta - abc : Subsystem
  d/q - alfa/beta : Subsystem
  Uabc_ref : Outport
  wires:
  d/q - alfa/beta/1(alfa/beta) -> alfa/beta - abc/1(alfa/beta)
  Ud/Uq/1 -> d/q - alfa/beta/1(d/q)
  alfa/beta - abc/1(abc) -> Uabc_ref/1
  theta/1 -> d/q - alfa/beta/2(tita)

== system Bitchplzwork/Wind 3 KW, 50HZ, 440V1/Pitch_angle-controller ==
  wr : Inport
  0-pitch_max : Saturate  UpperLimit=45  LowerLimit=0
  Constant2 : Constant  Value=2
  "Rate Limiter   " : RateLimiter  RisingSlewLimit=2  FallingSlewLimit=-2
  Sum : Sum  Inputs=|+-  SaturateOnIntegerOverflow=on
  genertaor terminal6 : Scope  NumInputPorts=2
  pitch_gain : Gain  Gain=500  SaturateOnIntegerOverflow=on  OutDataTypeStr=Inherit: Same as input  ParamDataTypeStr=Inherit: Same as input
  Pitch_angle : Outport
  wires:
  "Rate Limiter   "/1 -> Pitch_angle/1, genertaor terminal6/1
  pitch_gain/1 -> 0-pitch_max/1
  Sum/1 -> pitch_gain/1
  Constant2/1 -> Sum/2
  0-pitch_max/1 -> "Rate Limiter   "/1, genertaor terminal6/2
  wr/1 -> Sum/1

== system Bitchplzwork/Battery DC-DC converter /Battery Converter  Control/PI 1 ==
  e : Inport
  Gain1 : Gain  Gain=0.65
  Gain2 : Gain  Gain=150
  Integrator : Integrator
  Saturation : Saturate  UpperLimit=500  LowerLimit=-100
  Sum1 : Sum  Inputs=|++
  " " : Outport
  wires:
  Saturation/1 -> " "/1
  Gain2/1 -> Integrator/1
  e/1 -> Gain1/1, Gain2/1
  Gain1/1 -> Sum1/1
  Integrator/1 -> Sum1/2
  Sum1/1 -> Saturation/1

== system Bitchplzwork/Battery DC-DC converter /Battery Converter  Control/PI 2 ==
  e : Inport
  Gain1 : Gain
  Gain2 : Gain
  Integrator : Integrator
  Saturation : Saturate  UpperLimit=1  LowerLimit=-1
  Sum1 : Sum  Inputs=|++
  " " : Outport
  wires:
  Sum1/1 -> Saturation/1
  Integrator/1 -> Sum1/2
  Gain1/1 -> Sum1/1
  e/1 -> Gain2/1, Gain1/1
  Gain2/1 -> Integrator/1
  Saturation/1 -> " "/1

== system Bitchplzwork/Battery DC-DC converter /Battery Converter  Control/Subsystem1 ==
  Vdc_ref : Inport
  LPF vq6 : powerlib_extras/Discrete  Control Blocks/Discrete 1st-Order Filter  FilterType=Lowpass  Tc=10e-3  Ts=Tss  Initialize=off  Vac_Init=[0.8 -25 50]  Vdc_Init=0  PlotResponse=off  param1=[1 100 0.1]
      settings: SourceProductName=Simscape Electrical  SourceProductBaseCode=PS
  To Workspace1 : ToWorkspace  VariableName=Vdc_ref  SampleTime=-1
  wires:
  Vdc_ref/1 -> LPF vq6/1
  LPF vq6/1 -> [Vdc], To Workspace1/1

== system Bitchplzwork/Battery DC-DC converter /Battery Converter  Control/Subsystem2 ==
  Ibat_ref : Inport
  LPF vq6 : powerlib_extras/Discrete  Control Blocks/Discrete 1st-Order Filter  FilterType=Lowpass  Tc=10e-3  Ts=Tss  Initialize=off  Vac_Init=[0.8 -25 50]  Vdc_Init=0  PlotResponse=off  param1=[1 100 0.1]
      settings: SourceProductName=Simscape Electrical  SourceProductBaseCode=PS
  To Workspace1 : ToWorkspace  VariableName=Ibat_ref  SampleTime=-1
  tag scope: Ibat_ref=global
  wires:
  LPF vq6/1 -> To Workspace1/1, [Ibat_ref]
  Ibat_ref/1 -> LPF vq6/1

== system Bitchplzwork/Battery DC-DC converter /Battery Converter  Control/Subsystem3 ==
  ILbat : Inport
  LPF vq6 : powerlib_extras/Discrete  Control Blocks/Discrete 1st-Order Filter  FilterType=Lowpass  Tc=10e-3  Ts=Tss  Initialize=off  Vac_Init=[0.8 -25 50]  Vdc_Init=0  PlotResponse=off  param1=[1 100 0.1]
      settings: SourceProductName=Simscape Electrical  SourceProductBaseCode=PS
  To Workspace1 : ToWorkspace  VariableName=ILbat  SampleTime=-1
  wires:
  ILbat/1 -> LPF vq6/1
  LPF vq6/1 -> To Workspace1/1
